simulink subsystem "battery"  (R2024a)
settings: Solver=VariableStepAuto  StartTime=0.0  StopTime=10.0  RelTol=1e-3
model mask{initial_in_temp=0, initial_air_temp=0, initial_soc=0, initial_soh=0, t_alpha=0, t_beta=0, t_tref=0, ocv_v0=0, ocv_vl=0, ocv_alpha=0, ocv_beta=0, ocv_gamma=0, ehc_a=0, ehc_b=0, ehc_kappa=0, ehc_mu=0, ehc_sigma=0, ehc_lambda=0, th_cp=0, th_cair=0, th_rin=0, th_rout=0, th_rair=0}
  mask prompts: initial_in_temp "Initial internal temperature"; initial_air_temp "Initial air temperature"; initial_soc "Initial SoC"; initial_soh "Initial SoH"; t_alpha "α"; t_beta "β"; t_tref "Tref"; ocv_v0 "v0"; ocv_vl "vl"; ocv_alpha "α"; ocv_beta "β"; ocv_gamma "γ"; ehc_a "A"; ehc_b "B"; ehc_kappa "κ"; ehc_mu "μ"; ehc_sigma "σ"; ehc_lambda "λ"; th_cp "Cp"; th_cair "Cair"; th_rin "Rin"; th_rout "Rout"; th_rair "Rair"
undefined symbols (not defined in the file): COULOMBIC_EFFICIENCIES, INTERNAL_RESISTANCE, LOWER_VOLT_CF, NOMINAL_CAPACITY
libraries: fl_lib x9, nesl_utility x5, simulink x4, dspsigops x2, ee_lib x1
settings Model: Creator=Cristobal  LastModifiedBy=n0ne
settings ModelReferenceCC: EnableRefExpFcnMdlSchedulingChecks=on
settings RTWCC: GPUComputeCapability=3.5

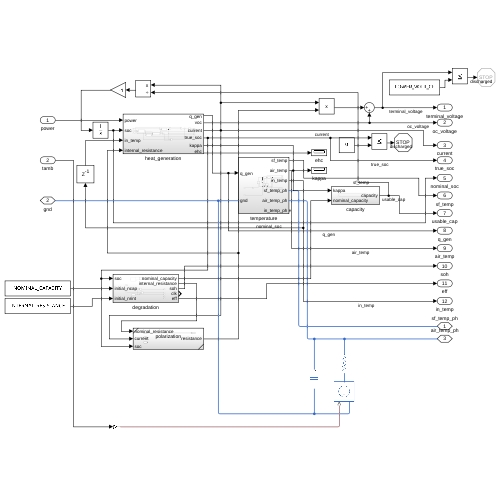
[thumbnail: Simulink's stored preview of the top-level diagram]
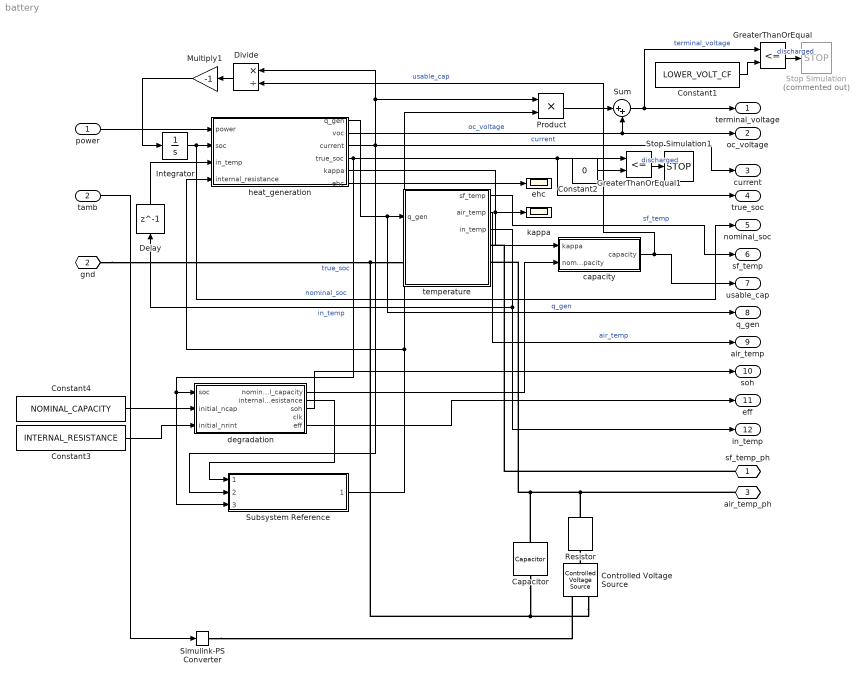
== system battery ==
  power : Inport
  tamb : Inport  Port=2
  Capacitor : fl_lib/Electrical/Electrical Elements/Capacitor  c=th_cair F  r=0 Ohm  g=0 1/Ohm  i_specify=off  i_priority=None  i=0 A  i_nominal_specify=off  i_nominal_value=1  i_nominal_unit=A  v_specify=off  v_priority=None  v=0 V  v_nominal_specify=off  v_nominal_value=1  v_nominal_unit=V  vc_specify=on  vc_priority=High  vc=initial_air_temp V  vc_nominal_specify=off  vc_nominal_value=1  vc_nominal_unit=V
  Constant1 : Constant  Value=LOWER_VOLT_CF
  Constant2 : Constant  Value=0
  Constant3 : Constant  Value=INTERNAL_RESISTANCE
  Constant4 : Constant  Value=NOMINAL_CAPACITY
  Controlled Voltage Source : fl_lib/Electrical/Electrical Sources/Controlled Voltage Source
  Delay : Delay  DelayLength=1  InitialCondition=initial_air_temp
  Divide : Product  Inputs=*/
  GreaterThanOrEqual : RelationalOperator  Operator=<=  OutDataTypeStr=boolean  RndMeth=Simplest  InputSameDT=off
  GreaterThanOrEqual1 : RelationalOperator  Operator=<=  OutDataTypeStr=boolean  RndMeth=Simplest  InputSameDT=off
  Integrator : Integrator  InitialCondition=initial_soc
  Multiply1 : Gain  Gain=-1
  Product : Product
  Resistor : fl_lib/Electrical/Electrical Elements/Resistor  R=th_rair Ohm  i_specify=off  i_priority=None  i=0 A  i_nominal_specify=off  i_nominal_value=1  i_nominal_unit=A  v_specify=off  v_priority=None  v=0 V  v_nominal_specify=off  v_nominal_value=1  v_nominal_unit=V
  Simulink-PS Converter : nesl_utility/Simulink-PS Converter  PhysicalDomain=network_engine_domain  SubClassName=ps_input  LeftPortType=input  RightPortType=output  PseudoPeriodic=off  Frequencies=[]  NoiseDistribution=none  NoiseParameters=[]  Unit=1  AffineConversion=off  FilteringAndDerivatives=provide  SimscapeFilterOrder=1  InputFilterTimeConstant=0.001  UdotUserProvided=0
  Stop Simulation : Stop  Commented=on
  Stop Simulation1 : Stop
  Subsystem Reference : Subsystem  ReferencedSubsystem=polarization
  Sum : Sum  Inputs=|++
  capacity : Subsystem
  degradation : Subsystem
  ehc : Scope
  heat_generation : Subsystem
  kappa : Scope
  temperature : Subsystem
  sf_temp_ph : PMIOPort  Side=Right
  gnd : PMIOPort  Port=2  Side=Left
  air_temp_ph : PMIOPort  Port=3  Side=Right
  terminal_voltage : Outport
  oc_voltage : Outport  Port=2
  current : Outport  Port=3
  true_soc : Outport  Port=4
  nominal_soc : Outport  Port=5
  sf_temp : Outport  Port=6
  usable_cap : Outport  Port=7
  q_gen : Outport  Port=8
  air_temp : Outport  Port=9
  soh : Outport  Port=10
  eff : Outport  Port=11
  in_temp : Outport  Port=12
  wires:
  temperature/1(sf_temp) -> sf_temp/1  "sf_temp"
  heat_generation/1(q_gen) -> temperature/1(q_gen), q_gen/1  "q_gen"
  capacity/1(capacity) -> Divide/2, usable_cap/1  "usable_cap"
  heat_generation/2(voc) -> Sum/2, oc_voltage/1  "oc_voltage"
  heat_generation/3(current) -> Subsystem Reference/2, Product/1, Divide/1, current/1  "current"
  Product/1 -> Sum/1
  Sum/1 -> GreaterThanOrEqual/1, terminal_voltage/1  "terminal_voltage"
  heat_generation/4(true_soc) -> Subsystem Reference/3, degradation/1(soc), true_soc/1, GreaterThanOrEqual1/1  "true_soc"
  Integrator/1 -> heat_generation/2(soc), nominal_soc/1  "nominal_soc"
  Divide/1 -> Multiply1/1
  Multiply1/1 -> Integrator/1
  Constant1/1 -> GreaterThanOrEqual/2
  power/1 -> heat_generation/1(power)
  GreaterThanOrEqual/1 -> Stop Simulation/1  "discharged"
  heat_generation/6(ehc) -> ehc/1
  temperature/2(air_temp) -> air_temp/1  "air_temp"
  GreaterThanOrEqual1/1 -> Stop Simulation1/1  "discharged"
  Constant2/1 -> GreaterThanOrEqual1/2
  Subsystem Reference/1 -> Product/2, heat_generation/4(internal_resistance)
  degradation/3(soh) -> soh/1
  degradation/1(nominal_capacity) -> capacity/2(nominal_capacity)
  degradation/5(eff) -> eff/1
  Constant4/1 -> degradation/2(initial_ncap)
  Constant3/1 -> degradation/3(initial_nrint)
  heat_generation/5(kappa) -> capacity/1(kappa), kappa/1
  Delay/1 -> heat_generation/3(in_temp)
  tamb/1 -> Simulink-PS Converter/1
  temperature/3(in_temp) -> in_temp/1, Delay/1  "in_temp"
  degradation/2(internal_resistance) -> Subsystem Reference/1
  connections:
  sf_temp_ph/RConn1 -- temperature/RConn1
  gnd/RConn1 -- Capacitor/RConn1 -- Controlled Voltage Source/RConn2 -- temperature/LConn1
  air_temp_ph/RConn1 -- Resistor/LConn1 -- Capacitor/LConn1 -- temperature/RConn2
  Controlled Voltage Source/LConn1 -- Resistor/RConn1
  Simulink-PS Converter/RConn1 -- Controlled Voltage Source/RConn1

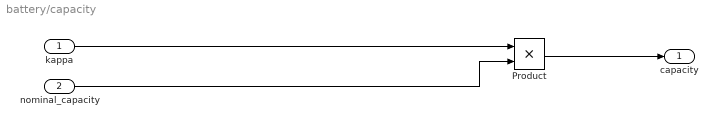
== system battery/capacity ==
  kappa : Inport
  nominal_capacity : Inport  Port=2
  Product : Product
  capacity : Outport
  wires:
  kappa/1 -> Product/1
  Product/1 -> capacity/1
  nominal_capacity/1 -> Product/2

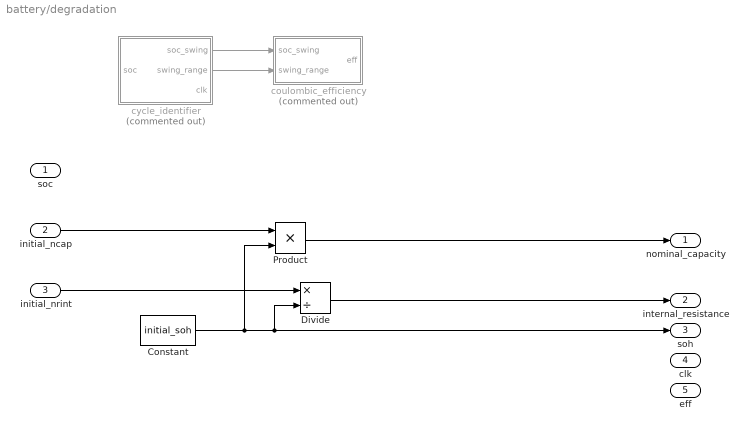
== system battery/degradation ==
  soc : Inport
  initial_ncap : Inport  Port=2
  initial_nrint : Inport  Port=3
  Constant : Constant  Value=initial_soh
  Divide : Product  Inputs=*/
  Product : Product
  coulombic_efficiency : Subsystem  Commented=on
  cycle_identifier : Subsystem  Commented=on
  nominal_capacity : Outport
  internal_resistance : Outport  Port=2
  soh : Outport  Port=3
  clk : Outport  Port=4
  eff : Outport  Port=5
  wires:
  Constant/1 -> Product/2, Divide/2, soh/1
  cycle_identifier/1(soc_swing) -> coulombic_efficiency/1(soc_swing)
  cycle_identifier/2(swing_range) -> coulombic_efficiency/2(swing_range)
  initial_ncap/1 -> Product/1
  Product/1 -> nominal_capacity/1
  initial_nrint/1 -> Divide/1
  Divide/1 -> internal_resistance/1

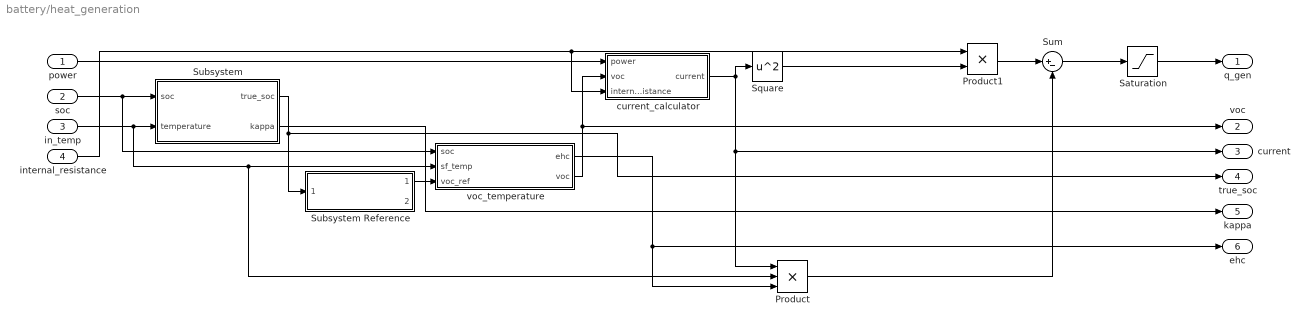
== system battery/heat_generation ==
  power : Inport
  soc : Inport  Port=2
  in_temp : Inport  Port=3
  internal_resistance : Inport  Port=4
  Product : Product  Inputs=3
  Product1 : Product
  Saturation : Saturate  UpperLimit=inf  LowerLimit=0
  Square : Math  Operator=square
  Subsystem : Subsystem
  Subsystem Reference : Subsystem  ReferencedSubsystem=voc
  Sum : Sum  Inputs=|+-
  current_calculator : Subsystem
  voc_temperature : Subsystem
  q_gen : Outport
  voc : Outport  Port=2
  current : Outport  Port=3
  true_soc : Outport  Port=4
  kappa : Outport  Port=5
  ehc : Outport  Port=6
  wires:
  Subsystem Reference/1 -> voc_temperature/3(voc_ref)
  voc_temperature/2(voc) -> current_calculator/2(voc), voc/1
  in_temp/1 -> Subsystem/2(temperature), voc_temperature/2(sf_temp), Product/2
  soc/1 -> voc_temperature/1(soc), Subsystem/1(soc)
  Subsystem/2(kappa) -> kappa/1
  power/1 -> current_calculator/1(power)
  current_calculator/1(current) -> current/1, Product/1, Square/1
  Square/1 -> Product1/2
  Product1/1 -> Sum/1
  voc_temperature/1(ehc) -> Product/3, ehc/1
  Product/1 -> Sum/2
  Subsystem/1(true_soc) -> true_soc/1, Subsystem Reference/1
  Sum/1 -> Saturation/1
  Saturation/1 -> q_gen/1
  internal_resistance/1 -> current_calculator/3(internal_resistance), Product1/1

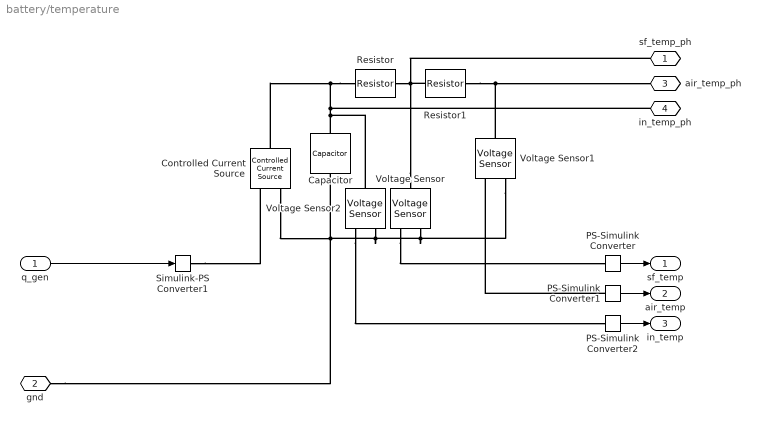
== system battery/temperature ==
  q_gen : Inport
  Capacitor : ee_lib/Passive/Capacitor  cap_option=ee.enum.passive.capacitor.capOption.const  c=th_cp F  Cvec=[1e-05, 1e-06] F  Vvec=[0, 10] V  CV_table_symmetry=1  f_vec=[1, 10] kHz  DFext_vec=[.8, 1.2]  enable_C_tol=0  averaging_period=0 s  C_tol=5  tol_distribution=1  nSigma=4  r=0 Ohm  g=0 1/Ohm  maxPermissibleTemperature=85 degC  tFailOnTemperature=1 s  enable_operating_limits=0  operating_limit_action=2  max_working_voltage_range=[-25, 25] V  power_rating=1 W  maxTemperature=85 degC  thermalEnable=false  thermalMass=1 J/K  enable_faults=ee.enum.enable.no  fault_action=simscape.enum.assert.action.none  Cscale_faulted=100  R_faulted=1e-3 Ohm  G_faulted=0 1/Ohm  tau_fault=1e-3 s  fault_trigger=ee.enum.faults.faultTrigger.temporal  t_fault=1 s  max_permissible_voltage_range=[-100, 100] V  t_fail_on_voltage=1 s  i_specify=off  i_priority=None  i=0 A  i_nominal_specify=off  i_nominal_value=1  i_nominal_unit=A  v_specify=off  v_priority=None  v=303 V  v_nominal_specify=off  v_nominal_value=1  v_nominal_unit=V  vc_specify=on  vc_priority=High  vc=initial_in_temp V  vc_nominal_specify=off  vc_nominal_value=1  vc_nominal_unit=V  T_specify=off  T_priority=None  T=298.15 K  T_nominal_specify=off  T_nominal_value=1  T_nominal_unit=K
  Controlled Current Source : fl_lib/Electrical/Electrical Sources/Controlled Current Source
  PS-Simulink Converter : nesl_utility/PS-Simulink Converter  PhysicalDomain=network_engine_domain  SubClassName=ps_output  LeftPortType=input  RightPortType=output  PseudoPeriodic=off  Frequencies=[]  VectorFormat=inherit  Unit=1  AffineConversion=off
  PS-Simulink Converter1 : nesl_utility/PS-Simulink Converter  PhysicalDomain=network_engine_domain  SubClassName=ps_output  LeftPortType=input  RightPortType=output  PseudoPeriodic=off  Frequencies=[]  VectorFormat=inherit  Unit=1  AffineConversion=off
  PS-Simulink Converter2 : nesl_utility/PS-Simulink Converter  PhysicalDomain=network_engine_domain  SubClassName=ps_output  LeftPortType=input  RightPortType=output  PseudoPeriodic=off  Frequencies=[]  VectorFormat=inherit  Unit=1  AffineConversion=off
  Resistor : fl_lib/Electrical/Electrical Elements/Resistor  R=th_rin Ohm  i_specify=off  i_priority=None  i=0 A  i_nominal_specify=off  i_nominal_value=1  i_nominal_unit=A  v_specify=off  v_priority=None  v=0 V  v_nominal_specify=off  v_nominal_value=1  v_nominal_unit=V
  Resistor1 : fl_lib/Electrical/Electrical Elements/Resistor  R=th_rout Ohm  i_specify=off  i_priority=None  i=0 A  i_nominal_specify=off  i_nominal_value=1  i_nominal_unit=A  v_specify=off  v_priority=None  v=0 V  v_nominal_specify=off  v_nominal_value=1  v_nominal_unit=V
  Simulink-PS Converter1 : nesl_utility/Simulink-PS Converter  PhysicalDomain=network_engine_domain  SubClassName=ps_input  LeftPortType=input  RightPortType=output  PseudoPeriodic=off  Frequencies=[]  NoiseDistribution=none  NoiseParameters=[]  Unit=1  AffineConversion=off  FilteringAndDerivatives=provide  SimscapeFilterOrder=1  InputFilterTimeConstant=0.001  UdotUserProvided=0
  Voltage Sensor : fl_lib/Electrical/Electrical Sensors/Voltage Sensor
  Voltage Sensor1 : fl_lib/Electrical/Electrical Sensors/Voltage Sensor
  Voltage Sensor2 : fl_lib/Electrical/Electrical Sensors/Voltage Sensor
  sf_temp_ph : PMIOPort  Side=Right
  gnd : PMIOPort  Port=2  Side=Left
  air_temp_ph : PMIOPort  Port=3  Side=Right
  in_temp_ph : PMIOPort  Port=4  Side=Right
  sf_temp : Outport
  air_temp : Outport  Port=2
  in_temp : Outport  Port=3
  wires:
  PS-Simulink Converter1/1 -> air_temp/1
  q_gen/1 -> Simulink-PS Converter1/1
  PS-Simulink Converter/1 -> sf_temp/1
  PS-Simulink Converter2/1 -> in_temp/1
  connections:
  PS-Simulink Converter1/LConn1 -- Voltage Sensor1/RConn1
  Voltage Sensor1/LConn1 -- Resistor1/RConn1 -- air_temp_ph/RConn1
  Voltage Sensor/LConn1 -- Resistor1/LConn1 -- Resistor/RConn1 -- sf_temp_ph/RConn1
  Voltage Sensor/RConn1 -- PS-Simulink Converter/LConn1
  Voltage Sensor1/RConn2 -- Voltage Sensor/RConn2 -- Voltage Sensor2/RConn2 -- gnd/RConn1 -- Capacitor/RConn1 -- Controlled Current Source/RConn2
  Resistor/LConn1 -- in_temp_ph/RConn1 -- Voltage Sensor2/LConn1 -- Capacitor/LConn1 -- Controlled Current Source/LConn1
  Simulink-PS Converter1/RConn1 -- Controlled Current Source/RConn1
  Voltage Sensor2/RConn1 -- PS-Simulink Converter2/LConn1

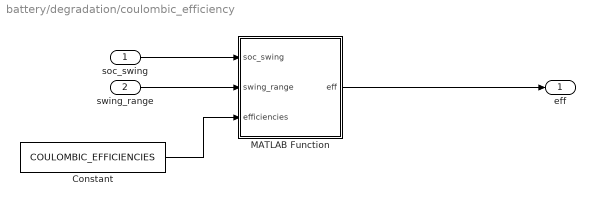
== system battery/degradation/coulombic_efficiency ==
  soc_swing : Inport
  swing_range : Inport  Port=2
  Constant : Constant  Value=COULOMBIC_EFFICIENCIES
  MATLAB Function : MATLAB Function  TreatAsAtomicUnit=on  SystemSampleTime=1
  eff : Outport
  wires:
  soc_swing/1 -> MATLAB Function/1(soc_swing)
  swing_range/1 -> MATLAB Function/2(swing_range)
  MATLAB Function/1(eff) -> eff/1
  Constant/1 -> MATLAB Function/3(efficiencies)

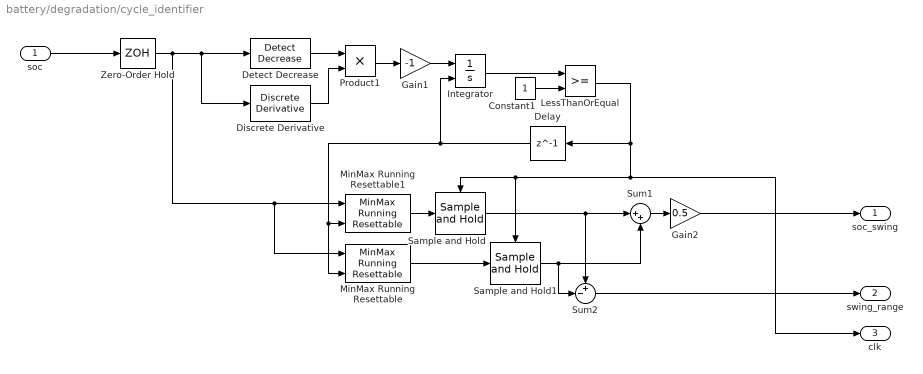
== system battery/degradation/cycle_identifier ==
  soc : Inport
  Constant1 : Constant
  Delay : Delay  DelayLength=1  SampleTime=1
  Detect Decrease : simulink/Logic and Bit Operations/Detect Decrease  vinit=0.0  OutDataTypeStr=boolean
  Discrete Derivative : simulink/Discrete/Discrete Derivative  gainval=1.0  ICPrevScaledInput=0.0  OutMin=[]  OutMax=[]  OutDataType=fixdt(1, 16)  OutScaling=2^-10  DoSatur=off
  Gain1 : Gain  Gain=-1
  Gain2 : Gain  Gain=0.5
  Integrator : Integrator  ExternalReset=rising
  LessThanOrEqual : RelationalOperator  OutDataTypeStr=boolean  RndMeth=Simplest  InputSameDT=off
  MinMax Running Resettable : simulink/Math Operations/MinMax Running Resettable  Function=min  vinit=1
  MinMax Running Resettable1 : simulink/Math Operations/MinMax Running Resettable  Function=max  vinit=0.0
  Product1 : Product
  Sample and Hold : dspsigops/Sample and Hold  trig=Rising edge  initCond=0  latchinput=off
  Sample and Hold1 : dspsigops/Sample and Hold  trig=Rising edge  initCond=0  latchinput=off
  Sum1 : Sum  Inputs=|++
  Sum2 : Sum  Inputs=+-|
  Zero-Order Hold : ZeroOrderHold
  soc_swing : Outport
  swing_range : Outport  Port=2
  clk : Outport  Port=3
  wires:
  Sum1/1 -> Gain2/1
  Gain2/1 -> soc_swing/1
  MinMax Running Resettable1/1 -> Sample and Hold/1
  Sample and Hold1/1 -> Sum1/2, Sum2/2
  Delay/1 -> MinMax Running Resettable/2, MinMax Running Resettable1/2, Integrator/2
  Constant1/1 -> LessThanOrEqual/2
  MinMax Running Resettable/1 -> Sample and Hold1/1
  Detect Decrease/1 -> Product1/1
  Product1/1 -> Gain1/1
  LessThanOrEqual/1 -> clk/1, Sample and Hold1/Trigger, Sample and Hold/Trigger, Delay/1
  Sample and Hold/1 -> Sum2/1, Sum1/1
  Gain1/1 -> Integrator/1
  Zero-Order Hold/1 -> MinMax Running Resettable/1, MinMax Running Resettable1/1, Discrete Derivative/1, Detect Decrease/1
  Integrator/1 -> LessThanOrEqual/1
  Discrete Derivative/1 -> Product1/2
  soc/1 -> Zero-Order Hold/1
  Sum2/1 -> swing_range/1

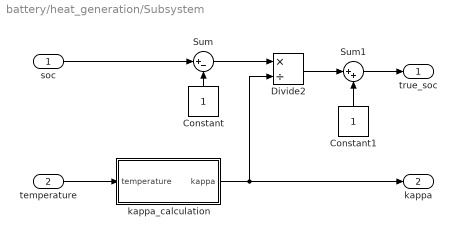
== system battery/heat_generation/Subsystem ==
  soc : Inport
  temperature : Inport  Port=2
  Constant : Constant
  Constant1 : Constant
  Divide2 : Product  Inputs=*/
  Sum : Sum  Inputs=|+-
  Sum1 : Sum  Inputs=|++
  kappa_calculation : Subsystem
  true_soc : Outport
  kappa : Outport  Port=2
  wires:
  Sum1/1 -> true_soc/1
  Constant1/1 -> Sum1/2
  Divide2/1 -> Sum1/1
  Sum/1 -> Divide2/1
  Constant/1 -> Sum/2
  soc/1 -> Sum/1
  temperature/1 -> kappa_calculation/1(temperature)
  kappa_calculation/1(kappa) -> kappa/1, Divide2/2

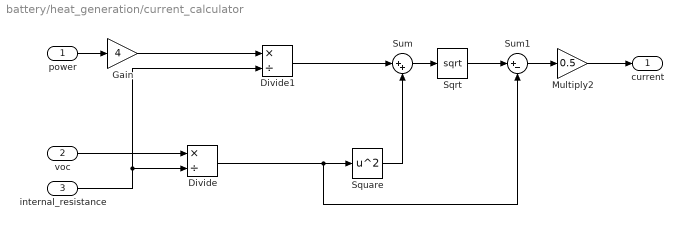
== system battery/heat_generation/current_calculator ==
  power : Inport
  voc : Inport  Port=2
  internal_resistance : Inport  Port=3
  Divide : Product  Inputs=*/
  Divide1 : Product  Inputs=*/
  Gain : Gain  Gain=4
  Multiply2 : Gain  Gain=0.5
  Sqrt : Sqrt
  Square : Math  Operator=square
  Sum : Sum  Inputs=|++
  Sum1 : Sum  Inputs=|+-
  current : Outport
  wires:
  power/1 -> Gain/1
  Divide1/1 -> Sum/1
  Divide/1 -> Sum1/2, Square/1
  Square/1 -> Sum/2
  Sum/1 -> Sqrt/1
  Sqrt/1 -> Sum1/1
  Sum1/1 -> Multiply2/1
  Multiply2/1 -> current/1
  voc/1 -> Divide/1
  internal_resistance/1 -> Divide/2, Divide1/2
  Gain/1 -> Divide1/1

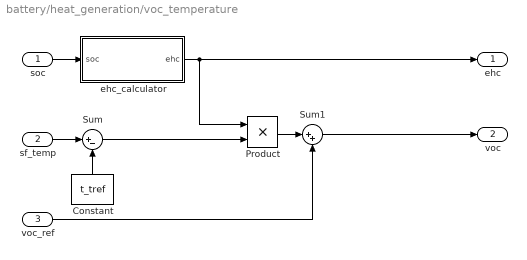
== system battery/heat_generation/voc_temperature ==
  soc : Inport
  sf_temp : Inport  Port=2
  voc_ref : Inport  Port=3
  Constant : Constant  Value=t_tref
  Product : Product
  Sum : Sum  Inputs=|+-
  Sum1 : Sum  Inputs=|++
  ehc_calculator : Subsystem
  ehc : Outport
  voc : Outport  Port=2
  wires:
  Sum1/1 -> voc/1
  voc_ref/1 -> Sum1/2
  Product/1 -> Sum1/1
  Sum/1 -> Product/2
  Constant/1 -> Sum/2
  sf_temp/1 -> Sum/1
  ehc_calculator/1(ehc) -> ehc/1, Product/1
  soc/1 -> ehc_calculator/1(soc)

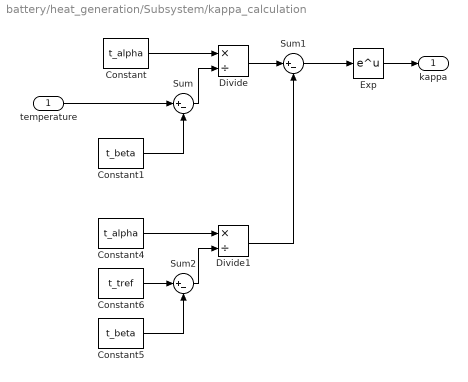
== system battery/heat_generation/Subsystem/kappa_calculation ==
  temperature : Inport
  Constant : Constant  Value=t_alpha
  Constant1 : Constant  Value=t_beta
  Constant4 : Constant  Value=t_alpha
  Constant5 : Constant  Value=t_beta
  Constant6 : Constant  Value=t_tref
  Divide : Product  Inputs=*/
  Divide1 : Product  Inputs=*/
  Exp : Math
  Sum : Sum  Inputs=|+-
  Sum1 : Sum  Inputs=|+-
  Sum2 : Sum  Inputs=|+-
  kappa : Outport
  wires:
  Exp/1 -> kappa/1
  temperature/1 -> Sum/1
  Divide1/1 -> Sum1/2
  Divide/1 -> Sum1/1
  Constant4/1 -> Divide1/1
  Constant/1 -> Divide/1
  Constant5/1 -> Sum2/2
  Constant1/1 -> Sum/2
  Sum/1 -> Divide/2
  Constant6/1 -> Sum2/1
  Sum1/1 -> Exp/1
  Sum2/1 -> Divide1/2

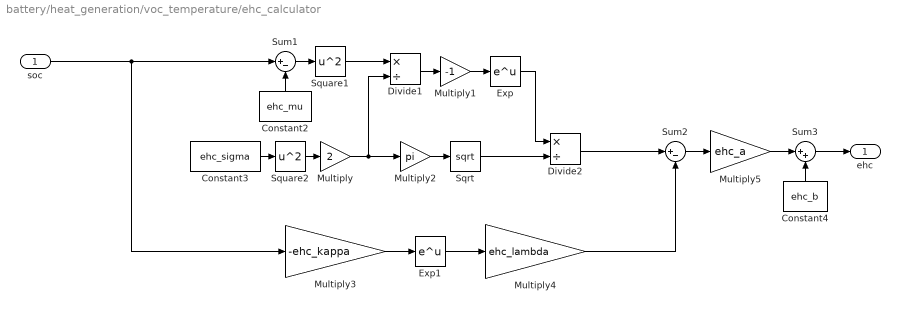
== system battery/heat_generation/voc_temperature/ehc_calculator ==
  soc : Inport
  Constant2 : Constant  Value=ehc_mu
  Constant3 : Constant  Value=ehc_sigma
  Constant4 : Constant  Value=ehc_b
  Divide1 : Product  Inputs=*/
  Divide2 : Product  Inputs=*/
  Exp : Math
  Exp1 : Math
  Multiply : Gain  Gain=2
  Multiply1 : Gain  Gain=-1
  Multiply2 : Gain  Gain=pi
  Multiply3 : Gain  Gain=-ehc_kappa
  Multiply4 : Gain  Gain=ehc_lambda
  Multiply5 : Gain  Gain=ehc_a
  Sqrt : Sqrt
  Square1 : Math  Operator=square
  Square2 : Math  Operator=square
  Sum1 : Sum  Inputs=|+-
  Sum2 : Sum  Inputs=|+-
  Sum3 : Sum  Inputs=|++
  ehc : Outport
  wires:
  Constant4/1 -> Sum3/2
  Divide2/1 -> Sum2/1
  Divide1/1 -> Multiply1/1
  Multiply2/1 -> Sqrt/1
  Multiply/1 -> Divide1/2, Multiply2/1
  Multiply1/1 -> Exp/1
  soc/1 -> Sum1/1, Multiply3/1
  Sum1/1 -> Square1/1
  Multiply5/1 -> Sum3/1
  Square2/1 -> Multiply/1
  Sqrt/1 -> Divide2/2
  Exp/1 -> Divide2/1
  Sum2/1 -> Multiply5/1
  Constant2/1 -> Sum1/2
  Square1/1 -> Divide1/1
  Exp1/1 -> Multiply4/1
  Sum3/1 -> ehc/1
  Constant3/1 -> Square2/1
  Multiply3/1 -> Exp1/1
  Multiply4/1 -> Sum2/2

== matlab function battery/degradation/coulombic_efficiency/MATLAB Function ==
  data: soc_swing input; eff output; swing_range input; efficiencies input
function eff = find_eff(soc_swing, swing_range, efficiencies)
X = efficiencies(:, [1, 2]);
Y = efficiencies(:, 3);
[idx, distances] = knnsearch(X, [soc_swing, swing_range], "K", 3);
inverse_distances = 1 ./ distances;
eff = inverse_distances * Y(idx) / sum(inverse_distances);
